simulink model "close_loop_step"  (R2017a)
settings: Solver=VariableStepAuto  StartTime=0.0  StopTime=T  RelTol=1e-3
values from neighbouring files (symbols this model uses):
  noise_amp = 1.0000e-07    (= 1e-07)    [close_loop_step_dg.m]    (also in open_loop_step_dg.m)
  seed = randi([0 1000],1)    [close_loop_step_dg.m]    (also in close_loop_tf2_dg.m; multi_sin_damp_dg.m; open_loop_step_dg.m; open_noise_dg.m)
  tau = 50    [testbench.m]
  Ts = 1/Fs    (= 0.01)    [close_loop_step_dg.m]    (also in close_loop_tf2_dg.m = 0.001; open_loop_step_dg.m; testbench.m)
libraries: simulink x3
settings Model: Creator=ljxia  LastModifiedBy=ljxia

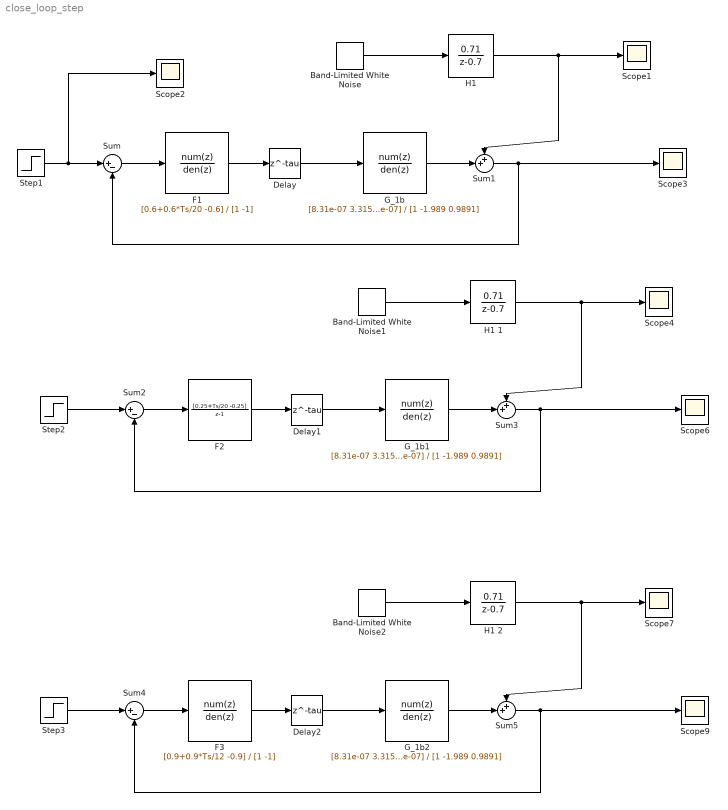
== system close_loop_step ==
  Band-Limited White Noise : simulink/Sources/Band-Limited White Noise  Cov=[noise_amp]  Ts=Ts  seed=[seed]
  Band-Limited White Noise1 : simulink/Sources/Band-Limited White Noise  Cov=[noise_amp]  Ts=Ts  seed=[seed]
  Band-Limited White Noise2 : simulink/Sources/Band-Limited White Noise  Cov=[noise_amp]  Ts=Ts  seed=[seed]
  Delay : Delay  DelayLength=tau  InitialCondition=0  SampleTime=Ts
  Delay1 : Delay  DelayLength=tau  InitialCondition=0  SampleTime=Ts
  Delay2 : Delay  DelayLength=tau  InitialCondition=0  SampleTime=Ts
  F1 : DiscreteTransferFcn  Numerator=[0.6+0.6*Ts/20 -0.6]  Denominator=[1 -1]  SampleTime=Ts
  F2 : DiscreteTransferFcn  Numerator=[0.25+Ts/20 -0.25]  Denominator=[1 -1]  SampleTime=Ts
  F3 : DiscreteTransferFcn  Numerator=[0.9+0.9*Ts/12 -0.9]  Denominator=[1 -1]  SampleTime=Ts
  G_1b : DiscreteTransferFcn  Numerator=[8.31e-07 3.315e-06 8.265e-07]  Denominator=[1 -1.989 0.9891]  SampleTime=Ts
  G_1b1 : DiscreteTransferFcn  Numerator=[8.31e-07 3.315e-06 8.265e-07]  Denominator=[1 -1.989 0.9891]  SampleTime=Ts
  G_1b2 : DiscreteTransferFcn  Numerator=[8.31e-07 3.315e-06 8.265e-07]  Denominator=[1 -1.989 0.9891]  SampleTime=Ts
  "H1 " : DiscreteTransferFcn  Numerator=[0.71]  Denominator=[1 -0.7]  SampleTime=Ts
  H1 1 : DiscreteTransferFcn  Numerator=[0.71]  Denominator=[1 -0.7]  SampleTime=Ts
  H1 2 : DiscreteTransferFcn  Numerator=[0.71]  Denominator=[1 -0.7]  SampleTime=Ts
  Scope{1..4,6..7,9} (7 alike) : Scope
  Step1 : Step  Time=0  SampleTime=0
  Step2 : Step  Time=0  SampleTime=0
  Step3 : Step  Time=0  SampleTime=0
  Sum : Sum  Inputs=|+-
  Sum1 : Sum  Inputs=++|
  Sum2 : Sum  Inputs=|+-
  Sum3 : Sum  Inputs=++|
  Sum4 : Sum  Inputs=|+-
  Sum5 : Sum  Inputs=++|
  wires:
  Delay/1 -> G_1b/1
  Step1/1 -> Scope2/1, Sum/1
  G_1b/1 -> Sum1/2
  Sum1/1 -> Sum/2, Scope3/1
  Sum/1 -> F1/1
  F1/1 -> Delay/1
  Band-Limited White Noise/1 -> "H1 "/1
  "H1 "/1 -> Sum1/1, Scope1/1
  Step2/1 -> Sum2/1
  Sum2/1 -> F2/1
  Delay1/1 -> G_1b1/1
  Sum3/1 -> Sum2/2, Scope6/1
  Band-Limited White Noise1/1 -> H1 1/1
  F2/1 -> Delay1/1
  G_1b1/1 -> Sum3/2
  H1 1/1 -> Sum3/1, Scope4/1
  Step3/1 -> Sum4/1
  Sum4/1 -> F3/1
  Delay2/1 -> G_1b2/1
  Sum5/1 -> Sum4/2, Scope9/1
  Band-Limited White Noise2/1 -> H1 2/1
  F3/1 -> Delay2/1
  G_1b2/1 -> Sum5/2
  H1 2/1 -> Sum5/1, Scope7/1
